simulink model "G_K"  (R2019a)
settings: Solver=VariableStepAuto  StartTime=0.0  StopTime=10.0  RelTol=1e-3
undefined symbols (not defined in the file): GKC_B, Q_gK, V_gK
settings Model: Creator=rache  LastModifiedBy=rache
settings DataIOCC: ReturnWorkspaceOutputs=off
settings DebuggingCC: ArithmeticOperatorsInVariantConditions=warning

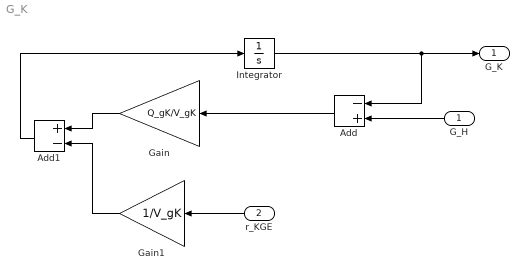
== system G_K ==
  G_H : Inport
  r_KGE : Inport  Port=2
  Add : Sum  Inputs=-+
  Add1 : Sum  Inputs=+-
  Gain : Gain  Gain=Q_gK/V_gK
  Gain1 : Gain  Gain=1/V_gK
  Integrator : Integrator  InitialCondition=GKC_B  LimitOutput=on  LowerSaturationLimit=0
  G_K : Outport
  wires:
  Integrator/1 -> Add/1, G_K/1
  G_H/1 -> Add/2
  Add/1 -> Gain/1
  Gain/1 -> Add1/1
  r_KGE/1 -> Gain1/1
  Gain1/1 -> Add1/2
  Add1/1 -> Integrator/1
